simulink model "afe_abc_inv_psm_2mods"  (R2025b)
settings: Solver=ode1be  StartTime=0.0  StopTime=simlength  FixedStep=tc  MaxStep=tc
undefined symbols (not defined in the file): Adrso, afe_pwm_phase_shift_mod1, Amplitude_U, Amplitude_V, Amplitude_W, Aresd, Bresd, Cresd, Crso, CTRPIFF_CLIP_RELEASE, dead_time_AFE, dead_time_INV, deepNEGeta, deepNEGxi, deepPOSxi, emf_fb_p, emf_fb_p_ccaller_1, emf_fb_p_ccaller_2, emf_p, emf_p_ccaller_1, emf_p_ccaller_2, end_time_LVRT, fPWM_AFE, fPWM_INV, g0_161Hz, g0_500Hz, g1_161Hz, g1_500Hz, i_grid_neg_eta_lim, i_grid_neg_eta_red_lim, i_grid_neg_xi_lim, i_grid_neg_xi_red_lim, i_grid_pos_eta_lim, i_grid_pos_eta_red_lim, ibez, id_lim, ieta_neg_ref_lim, ieta_pos_ref_lim, Igrid_phase_normalization_factor, inv_pwm_phase_shift_mod1, iq_lim, ixi_pos_ref_lim, k_frt_ref, kg, ki_afe, ki_i, ki_rc_neg_grid, ki_rc_pos_grid, ki_vs, ki_w, kp_afe, kp_i, kp_rc_neg_grid, kp_rc_pos_grid, kp_vs, kp_w, kw, l1, l2, La ... (+54)
libraries: fl_lib x116, nesl_utility x62, cstblocks x14, simulink x11, single_phase_transformer_lib x3, threephase_inductor_lib x2, flexshaft_lib x1, psm x1
(part 5 of 9)

== system afe_abc_inv_psm_2mods/afe_abc_inv_psm_mod1/AFE_control/afe_control/grid_voltage_phase_lock_loops/dq_pll_ccaller ==
  ug_abc_pu : Inport
  Bus Selector : BusSelector  OutputSignals=omega_pu_hat,gamma_hat,u_grid_xi,u_grid_eta,dqpll_pll_state
  C Caller : CCaller  FunctionName=dqpll_grid_process_simulink  PortSpecificationStruct="%)30     .    N H   8    (     @         %    \"     8    !     0         %  0 \"0    $    _    07)G3F%M90  4&]R=$YA;64 4V-O<&4     26YD97@     5'EP90      4VEZ90      27-';&]B86P   X    P    !@    @    $          4    (     0    ,    !         !   P!O=70 #@   #     &    \"     0         !0    @    !     P    $         $  # &]U=  .    .     8    (    !          %    \"     $    &     0         0   ...(+3319 chars)"
  Constant : Constant  Value=ts_afe
  Data Type Conversion{1..2,4..5} (4 alike) : DataTypeConversion  OutDataTypeStr=single  SaturateOnIntegerOverflow=off  RndMeth=Floor
  Data Type Conversion{6..10} (5 alike) : DataTypeConversion  OutDataTypeStr=double  SaturateOnIntegerOverflow=off  RndMeth=Floor
  Data Type Conversion3 : DataTypeConversion  OutDataTypeStr=uint8  SaturateOnIntegerOverflow=off  RndMeth=Floor
  Demux : Demux  Outputs=3
  Quantizer1 : Quantizer  QuantizationInterval=adc_quantization
  Quantizer2 : Quantizer  QuantizationInterval=adc_quantization
  Quantizer4 : Quantizer  QuantizationInterval=adc_quantization
  Step : Step  Time=0.01  Before=1  After=0
  Unit Delay1 : UnitDelay  SampleTime=-1  HasFrameUpgradeWarning=on
  Unit Delay2 : UnitDelay  SampleTime=-1  HasFrameUpgradeWarning=on
  Unit Delay3 : UnitDelay  SampleTime=-1  HasFrameUpgradeWarning=on
  first_harmonic_tracker : Scope  NumInputPorts=3
      settings: ActiveDisplayYMinimum=-1.8038768619298935  ActiveDisplayYMaximum=1.5708545297384262
  first_harmonic_tracker_phase_u : Subsystem
  first_harmonic_tracker_phase_v : Subsystem
  first_harmonic_tracker_phase_w : Subsystem
  gamma_hat : Outport  VectorParamsAs1DForOutWhenUnconnected=off
  omega_pu_hat : Outport  Port=2  VectorParamsAs1DForOutWhenUnconnected=off
  dqpll_uxi : Outport  Port=3  VectorParamsAs1DForOutWhenUnconnected=off
  dqpll_ueta : Outport  Port=4  VectorParamsAs1DForOutWhenUnconnected=off
  dqpll_state : Outport  Port=5  VectorParamsAs1DForOutWhenUnconnected=off
  wires:
  Step/1 -> Data Type Conversion3/1
  Constant/1 -> Data Type Conversion1/1
  Data Type Conversion3/1 -> C Caller/1
  Data Type Conversion2/1 -> C Caller/2
  Data Type Conversion4/1 -> C Caller/3
  Data Type Conversion5/1 -> C Caller/4
  Data Type Conversion1/1 -> C Caller/5
  C Caller/1 -> Bus Selector/1
  Bus Selector/1 -> Data Type Conversion6/1  "<omega_pu_hat>"
  Bus Selector/2 -> Data Type Conversion7/1  "<gamma_hat>"
  Bus Selector/3 -> Data Type Conversion8/1  "<u_grid_xi>"
  Bus Selector/4 -> Data Type Conversion9/1  "<u_grid_eta>"
  Bus Selector/5 -> Data Type Conversion10/1  "<dqpll_pll_state>"
  Data Type Conversion7/1 -> gamma_hat/1
  Data Type Conversion10/1 -> dqpll_state/1
  Data Type Conversion8/1 -> dqpll_uxi/1
  Data Type Conversion9/1 -> dqpll_ueta/1
  ug_abc_pu/1 -> Demux/1
  Demux/2 -> Quantizer1/1
  Demux/1 -> Quantizer2/1
  Demux/3 -> Quantizer4/1
  Quantizer2/1 -> Unit Delay2/1
  Unit Delay2/1 -> first_harmonic_tracker_phase_u/1(u)
  Unit Delay1/1 -> first_harmonic_tracker_phase_v/1(u)
  Unit Delay3/1 -> first_harmonic_tracker_phase_w/1(u)
  Quantizer1/1 -> Unit Delay1/1
  Quantizer4/1 -> Unit Delay3/1
  Data Type Conversion6/1 -> omega_pu_hat/1
  first_harmonic_tracker_phase_u/1(u_hat) -> first_harmonic_tracker/1, Data Type Conversion2/1  "tracker_phase_u"
  first_harmonic_tracker_phase_v/1(u_hat) -> first_harmonic_tracker/2, Data Type Conversion4/1  "tracker_phase_v"
  first_harmonic_tracker_phase_w/1(u_hat) -> first_harmonic_tracker/3, Data Type Conversion5/1  "tracker_phase_w"

== system afe_abc_inv_psm_2mods/afe_abc_inv_psm_mod1/AFE_control/afe_control/grid_voltage_sequences/grid_voltage_sampling_and_alpha_beta_transformation ==
  v_abc : Inport
  Demux : Demux  Outputs=3
  Mux : Mux  Inputs=3
  sample_hold_normalization : Subsystem
  v_abc2alphabeta : MATLAB Function  TreatAsAtomicUnit=on
  u_grid_alpha : Outport
  u_grid_beta : Outport  Port=2
  tag scope: vg_abc_pu_mod1=global
  wires:
  v_abc2alphabeta/1(alpha) -> u_grid_alpha/1  "u_grid_alpha"
  v_abc2alphabeta/2(beta) -> u_grid_beta/1  "u_grid_beta"
  Demux/1 -> sample_hold_normalization/1(vg_a)
  v_abc/1 -> Demux/1
  Demux/3 -> sample_hold_normalization/3(vg_c)
  Demux/2 -> sample_hold_normalization/2(vg_b)
  sample_hold_normalization/1(vg_a_pu) -> Mux/1
  sample_hold_normalization/2(vg_b_pu) -> Mux/2
  sample_hold_normalization/3(vg_c_pu) -> Mux/3
  Mux/1 -> [vg_abc_pu_mod1], v_abc2alphabeta/1(v_abc)

== system afe_abc_inv_psm_2mods/afe_abc_inv_psm_mod1/AFE_control/afe_control/grid_voltage_sequences/v_alphabeta2xieta ==
  alpha : Inport
  beta : Inport  Port=2
  gamma : Inport  Port=3
  MATLAB Function : MATLAB Function  TreatAsAtomicUnit=on
  MATLAB Function1 : MATLAB Function  TreatAsAtomicUnit=on
  xi : Outport
  eta : Outport  Port=2
  v_grid_neg_xi : Outport  Port=3
  v_grid_neg_eta : Outport  Port=4
  wires:
  alpha/1 -> MATLAB Function1/1(alpha), MATLAB Function/1(alpha)  "u_grid_alpha"
  beta/1 -> MATLAB Function1/2(beta), MATLAB Function/2(beta)  "u_grid_beta"
  gamma/1 -> MATLAB Function1/3(gamma), MATLAB Function/3(gamma)  "gamma_grid"
  MATLAB Function/1(xi) -> xi/1  "u_grid_pos_xi"
  MATLAB Function/2(eta) -> eta/1  "u_grid_pos_eta"
  MATLAB Function1/1(xi) -> v_grid_neg_xi/1  "u_grid_neg_xi"
  MATLAB Function1/2(eta) -> v_grid_neg_eta/1  "u_grid_neg_eta"

== system afe_abc_inv_psm_2mods/afe_abc_inv_psm_mod1/AFE_control/afe_control/grid_voltage_sequences/voltage_sequence_avg ==
  v_grid_pos_xi : Inport
  v_grid_pos_eta : Inport  Port=2
  v_grid_neg_xi : Inport  Port=3
  v_grid_neg_eta : Inport  Port=4
  Variant Source{1..4} (4 alike) : VariantSource  VariantControls={use_moving_average_from_ccaller_mod1 == 1, use_moving_average_from_ccaller_mod1 == 0}
  average_filter_ccaller : Subsystem
  average_filter_simulink : Subsystem
  v_grid_pos_xi_avg : Outport
  v_grid_pos_eta_avg : Outport  Port=2
  v_grid_neg_xi_avg : Outport  Port=3
  v_grid_neg_eta_avg : Outport  Port=4
  wires:
  v_grid_pos_xi/1 -> average_filter_simulink/1(v_grid_pos_xi), average_filter_ccaller/1(v_grid_pos_xi)
  v_grid_pos_eta/1 -> average_filter_simulink/2(v_grid_pos_eta), average_filter_ccaller/2(v_grid_pos_eta)
  v_grid_neg_xi/1 -> average_filter_simulink/3(v_grid_neg_xi), average_filter_ccaller/3(v_grid_neg_xi)
  v_grid_neg_eta/1 -> average_filter_simulink/4(v_grid_neg_eta), average_filter_ccaller/4(v_grid_neg_eta)
  Variant Source4/1 -> v_grid_pos_xi_avg/1
  Variant Source1/1 -> v_grid_pos_eta_avg/1
  Variant Source2/1 -> v_grid_neg_xi_avg/1
  Variant Source3/1 -> v_grid_neg_eta_avg/1
  average_filter_ccaller/1(v_grid_pos_xi_avg) -> Variant Source4/1
  average_filter_ccaller/2(v_grid_pos_eta_avg) -> Variant Source1/1
  average_filter_ccaller/3(v_grid_neg_xi_avg) -> Variant Source2/1
  average_filter_ccaller/4(v_grid_neg_eta_avg) -> Variant Source3/1
  average_filter_simulink/1(v_grid_pos_xi_avg) -> Variant Source4/2
  average_filter_simulink/2(v_grid_pos_eta_avg) -> Variant Source1/2
  average_filter_simulink/3(v_grid_neg_xi_avg) -> Variant Source2/2
  average_filter_simulink/4(v_grid_neg_eta_avg) -> Variant Source3/2

== system afe_abc_inv_psm_2mods/afe_abc_inv_psm_mod1/INV_control/inverter_control/current_ctrl/bemf_observer ==
  ialpha_pu : Inport
  ibeta_pu : Inport  Port=2
  ualpha_pu : Inport  Port=3
  ubeta_pu : Inport  Port=4
  udc_pu : Inport  Port=5
  BEMF Observer simulink/Ccaller : Scope  NumInputPorts=2
      settings: ActiveDisplayYMinimum=-0.30362  ActiveDisplayYMaximum=1.18723
  Mux : Mux  Inputs=3
  Mux1 : Mux  Inputs=3
  Variant Source : VariantSource  VariantControls={use_observer_from_simulink_module_1 == 1, use_observer_from_ccaller_module_1 == 1}
  Variant Source1 : VariantSource  VariantControls={use_observer_from_simulink_module_1 == 1, use_observer_from_ccaller_module_1 == 1}
  bemf_observer : Subsystem
  bemf_observer_ccaller : Subsystem
  phase_fault : Subsystem  Commented=on
  tag scope: omega_hat_pu_mod1=global, theta_hat_mod1=global
  wires:
  ialpha_pu/1 -> bemf_observer/1(ialpha_pu), bemf_observer_ccaller/1(ialpha_pu)
  ibeta_pu/1 -> bemf_observer_ccaller/2(ibeta_pu), bemf_observer/2(ibeta_pu)
  Mux/1 -> BEMF Observer simulink/Ccaller/1
  Mux1/1 -> BEMF Observer simulink/Ccaller/2
  ualpha_pu/1 -> bemf_observer_ccaller/3(ualpha_pu), bemf_observer/3(ualpha_pu)
  ubeta_pu/1 -> bemf_observer_ccaller/4(ubeta_pu), bemf_observer/4(ubeta_pu)
  bemf_observer/1(omega_pu) -> Variant Source/1, Mux/1  "omega_pu"
  bemf_observer_ccaller/2(theta_hat) -> Mux1/2, Variant Source1/2  "theta_hat_code"
  bemf_observer_ccaller/1(omega_pu) -> Mux/2, Variant Source/2  "omega_pu_code"
  bemf_observer/2(theta_hat) -> Variant Source1/1, Mux1/1  "theta_hat"
  Variant Source1/1 -> [theta_hat_mod1]
  Variant Source/1 -> [omega_hat_pu_mod1]
  phase_fault/1(omega_pu_encoder) -> Mux/3
  phase_fault/2(theta_hat_encoder) -> Mux1/3
  udc_pu/1 -> bemf_observer_ccaller/5(udc_pu), bemf_observer/5(udc_pu)

== system afe_abc_inv_psm_2mods/afe_abc_inv_psm_mod1/INV_control/inverter_control/current_ctrl/current_ctrl ==
  iq_ref : Inport
  udc_pu : Inport  Port=2
  MTPA _mod1 : Subsystem
  Sqrt : Sqrt
  Square : Math  Operator=square
  Square1 : Math  Operator=square
  Sum : Sum  Inputs=|++
  dq_pi_with_vector_antiwindup mod1 : Subsystem
  id_ref _mod1 : Subsystem
      settings: PortSchema="{\"entries\":[{\"content\":{\"sides\":[{\"content\":{},\"type\":\"ConnectorPlacement.EquallySpacedRectSide\",\"uuid\":\"42af5d69-f0eb-42c6-9e03-28c1d0757323\"},{\"content\":{\"connectorIds\":[\"Out1\"],\"side\":\"RIGHT\"},\"type\":\"ConnectorPlacement.EquallySpacedRectSide\",\"uuid\":\"dd68a9f9-d15f-4e57-9d9e-130889a7b90c\"},{\"content\":{\"connectorIds\":[\"In1\"],\"side\":\"TOP\"},\"type\":\"ConnectorPlacement.EquallySpacedRectSide\",\"uuid\":\"68c797a2-8439-4b8d-8368-b7485adf0676\"}]},\"type\":\"ConnectorPlacement.EquallySpacedConnector\",\"uuid\":\"693c5f1c-0580-4626-8f13-b27865dfb3ac\"}],\"packageUris\":[\"http://schema.mathworks.com/mf0/Connector/R2020b\"],\"version\":\"1.0\"}"
  idref/id mod1 : Scope  NumInputPorts=2
      settings: ActiveDisplayYMinimum=-0.56823  ActiveDisplayYMaximum=0.06368
  iqref/iq mod1 : Scope  NumInputPorts=2
      settings: ActiveDisplayYMinimum=-1.15343  ActiveDisplayYMaximum=0.24986  DataLoggingVariableName=ScopeData2
  ud : Outport
  uq : Outport  Port=2
  tag scope: id_pu_ref_mod1=global, iq_pu_ref_mod1=global, u_mot_pu_sim_mod1=global, ud_pu_sim_mod1=global, uq_pu_sim_mod1=global
  wires:
  [iq_pu_mod1] -> iqref/iq mod1/2, dq_pi_with_vector_antiwindup mod1/4(iq)  "iq"
  [id_pu_mod1] -> idref/id mod1/2, dq_pi_with_vector_antiwindup mod1/2(id)  "id"
  MTPA _mod1/1(Id_ref_mtpa) -> id_ref _mod1/1(id_mtpa), [id_pu_ref_mod1]  "id_ref"
  iq_ref/1 -> MTPA _mod1/1(iq_ref), iqref/iq mod1/1, dq_pi_with_vector_antiwindup mod1/3(iq_ref), [iq_pu_ref_mod1]  "iq_ref"
  dq_pi_with_vector_antiwindup mod1/1(ctrl_d_u) -> ud/1, [ud_pu_sim_mod1], Square1/1
  dq_pi_with_vector_antiwindup mod1/2(ctrl_q_u) -> uq/1, [uq_pu_sim_mod1], Square/1
  Square/1 -> Sum/1
  Sum/1 -> Sqrt/1
  Square1/1 -> Sum/2
  Sqrt/1 -> [u_mot_pu_sim_mod1]
  id_ref _mod1/1(id_ref) -> idref/id mod1/1, dq_pi_with_vector_antiwindup mod1/1(id_ref)
  udc_pu/1 -> dq_pi_with_vector_antiwindup mod1/5(udc_pu)

== system afe_abc_inv_psm_2mods/afe_abc_inv_psm_mod1/INV_control/inverter_control/current_ctrl/current_transformation ==
  u : Inport
  v : Inport  Port=2
  w : Inport  Port=3
  alphabeta2dq : MATLAB Function  TreatAsAtomicUnit=on
  uvw2alphabeta : MATLAB Function  TreatAsAtomicUnit=on
  tag scope: ialpha_pu_mod1=global, ibeta_pu_mod1=global, id_pu_mod1=global, iq_pu_mod1=global
  wires:
  w/1 -> uvw2alphabeta/3(w)
  alphabeta2dq/2(q) -> [iq_pu_mod1]  "iq_pu"
  alphabeta2dq/1(d) -> [id_pu_mod1]  "id_pu"
  v/1 -> uvw2alphabeta/2(v)
  uvw2alphabeta/2(beta) -> [ibeta_pu_mod1], alphabeta2dq/2(beta)  "ibeta_pu"
  uvw2alphabeta/1(alpha) -> [ialpha_pu_mod1], alphabeta2dq/1(alpha)  "ialpha_pu"
  [theta_hat_mod1] -> alphabeta2dq/3(gamma)
  u/1 -> uvw2alphabeta/1(u)

== system afe_abc_inv_psm_2mods/afe_abc_inv_psm_mod1/INV_control/inverter_control/current_ctrl/sample_hold_normalization ==
  iu : Inport
  iv : Inport  Port=2
  iw : Inport  Port=3
  Gain3 : Gain  Gain=-1
  Gain4 : Gain  Gain=-1
  Gain5 : Gain  Gain=-1
  Quantizer1 : Quantizer  QuantizationInterval=adc_quantization
  Quantizer2 : Quantizer  QuantizationInterval=adc_quantization
  Quantizer4 : Quantizer  QuantizationInterval=adc_quantization
  Unit Delay : UnitDelay  SampleTime=-1  HasFrameUpgradeWarning=on
  Unit Delay1 : UnitDelay  SampleTime=-1  HasFrameUpgradeWarning=on
  Unit Delay4 : UnitDelay  SampleTime=-1  HasFrameUpgradeWarning=on
  iu_pu : Outport
  iv_pu : Outport  Port=2
  iw_pu : Outport  Port=3
  wires:
  Unit Delay4/1 -> Gain5/1
  Unit Delay1/1 -> Gain4/1
  Unit Delay/1 -> Gain3/1
  Quantizer4/1 -> Unit Delay/1
  Quantizer1/1 -> Unit Delay1/1
  Quantizer2/1 -> Unit Delay4/1
  iu/1 -> Quantizer4/1
  iv/1 -> Quantizer1/1
  iw/1 -> Quantizer2/1
  Gain3/1 -> iu_pu/1
  Gain4/1 -> iv_pu/1
  Gain5/1 -> iw_pu/1

== system afe_abc_inv_psm_2mods/afe_abc_inv_psm_mod1/afe/sv_pwm/modulator1/PWM generator ==
  time_source : Inport
  phase : Inport  Port=2
  m_uvw() : Inport  Port=3
  Constant8 : Constant  Value=tc
  Constant9 : Constant  Value=f
  MATLAB Function : MATLAB Function  TreatAsAtomicUnit=on  SystemSampleTime=tc
  MATLAB Function1 : MATLAB Function  TreatAsAtomicUnit=on  SystemSampleTime=tc
  gate commands : Subsystem
  period : Constant  Value=1/f
  trgo : Outport
  gate_cmds : Outport  Port=2
  wires:
  period/1 -> MATLAB Function/3(period)
  phase/1 -> MATLAB Function/2(phase)
  MATLAB Function/1(y) -> gate commands/1(ramp_up_down), MATLAB Function1/3(ramp_up_down)
  MATLAB Function1/1(trgo) -> trgo/1
  Constant8/1 -> MATLAB Function1/1(sampling_time)
  Constant9/1 -> MATLAB Function1/2(fPWM)
  m_uvw()/1 -> gate commands/2(m_uvw())
  gate commands/1(gate_cmds) -> gate_cmds/1
  time_source/1 -> MATLAB Function/1(t)

== system afe_abc_inv_psm_2mods/afe_abc_inv_psm_mod1/inverter/inverter/sv_pwm/modulator1 ==
  u : Inport
  v : Inport  Port=2
  w : Inport  Port=3
  phase : Inport  Port=4
  Bus Creator : BusCreator  Inputs=3
  PWM generator : Subsystem  mask{f=fPWM_INV, m_up=0.98, m_low=0.02, dead_time=dead_time_INV, pos_cmd_gate=15, neg_cmd_gate=-10, polarity=1, tc=tc}
      mask prompts: f "Frequency (Hz)"; m_up "Max Input Modulation Value"; m_low "Min Input Modulation Value"; dead_time "Dead Time (s)"; pos_cmd_gate "Positive Gate Voltage (V)"; neg_cmd_gate "Negative Gate Voltage (V)"; polarity "Polarity (pu)"; tc "Sampling time"
  gate_cmds : Outport
  tag scope: TRGO_inv_module_1=global
  wires:
  [time_inv_module_1] -> PWM generator/1(time_source)
  Bus Creator/1 -> PWM generator/3(m_uvw())
  PWM generator/1(trgo) -> [TRGO_inv_module_1]
  u/1 -> Bus Creator/1
  v/1 -> Bus Creator/2
  w/1 -> Bus Creator/3
  phase/1 -> PWM generator/2(phase)
  PWM generator/2(gate_cmds) -> gate_cmds/1

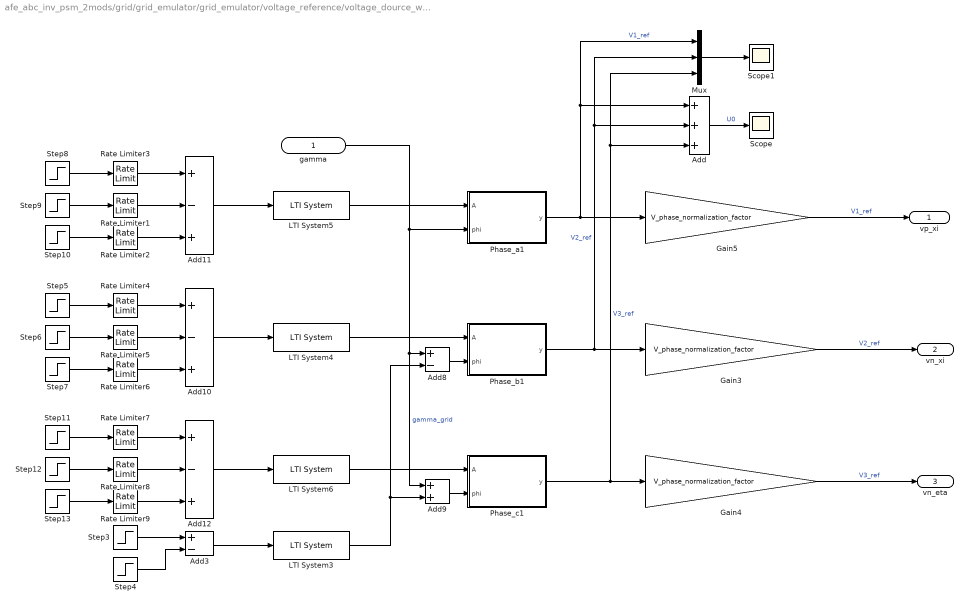
== system afe_abc_inv_psm_2mods/grid/grid_emulator/grid_emulator/voltage_reference/voltage_dource_with_frt ==
  gamma : Inport
  Add : Sum  Inputs=+++
  Add10 : Sum  Inputs=+-+
  Add11 : Sum  Inputs=+-+
  Add12 : Sum  Inputs=+-+
  Add3 : Sum  Inputs=+-
  Add8 : Sum  Inputs=+-
  Add9 : Sum
  Gain3 : Gain  Gain=V_phase_normalization_factor
  Gain4 : Gain  Gain=V_phase_normalization_factor
  Gain5 : Gain  Gain=V_phase_normalization_factor
  LTI System{3..6} (4 alike) : cstblocks/LTI System  sys=LVRT_flt_ss_c  IC=[0]  PadeOrder=0
  Mux : Mux  Inputs=3
  Phase_a1 : MATLAB Function  TreatAsAtomicUnit=on
  Phase_b1 : MATLAB Function  TreatAsAtomicUnit=on
  Phase_c1 : MATLAB Function  TreatAsAtomicUnit=on
  Rate Limiter{1..9} (9 alike) : RateLimiter  RisingSlewLimit=Vemu_ref_norm/t_ramp  FallingSlewLimit=-Vemu_ref_norm/t_ramp  SampleTimeMode=inherited
  Scope : Scope
      settings: ActiveDisplayYMinimum=-1E-15  ActiveDisplayYMaximum=8E-16
  Scope1 : Scope
      settings: ActiveDisplayYMinimum=-1.25511  ActiveDisplayYMaximum=1.25511
  Step10 : Step  Time=end_time_LVRT  After=Vemu_ref_norm*(1-Amplitude_U)  SampleTime=0
  Step11 : Step  Time=0  After=Vemu_ref_norm  SampleTime=0
  Step12 : Step  Time=start_time_LVRT  After=Vemu_ref_norm*(1-Amplitude_W)  SampleTime=0
  Step13 : Step  Time=end_time_LVRT  After=Vemu_ref_norm*(1-Amplitude_W)  SampleTime=0
  Step3 : Step  Time=start_time_LVRT  After=Phase_shift  SampleTime=0
  Step4 : Step  Time=end_time_LVRT  After=Phase_shift  SampleTime=0
  Step5 : Step  Time=0  After=Vemu_ref_norm  SampleTime=0
  Step6 : Step  Time=start_time_LVRT  After=Vemu_ref_norm*(1-Amplitude_V)  SampleTime=0
  Step7 : Step  Time=end_time_LVRT  After=Vemu_ref_norm*(1-Amplitude_V)  SampleTime=0
  Step8 : Step  Time=0  After=Vemu_ref_norm  SampleTime=0
  Step9 : Step  Time=start_time_LVRT  After=Vemu_ref_norm*(1-Amplitude_U)  SampleTime=0
  vp_xi : Outport  VectorParamsAs1DForOutWhenUnconnected=off
  vn_xi : Outport  Port=2  VectorParamsAs1DForOutWhenUnconnected=off
  vn_eta : Outport  Port=3  VectorParamsAs1DForOutWhenUnconnected=off
  wires:
  Phase_c1/1(y) -> Mux/3, Add/3, Gain4/1  "V3_ref"
  LTI System6/1 -> Phase_c1/1(A)
  gamma/1 -> Add9/1, Add8/1, Phase_a1/2(phi)  "gamma_grid"
  Add9/1 -> Phase_c1/2(phi)
  Add8/1 -> Phase_b1/2(phi)
  Phase_b1/1(y) -> Mux/2, Add/2, Gain3/1  "V2_ref"
  Phase_a1/1(y) -> Mux/1, Add/1, Gain5/1  "V1_ref"
  LTI System4/1 -> Phase_b1/1(A)
  Step5/1 -> Rate Limiter4/1
  Step6/1 -> Rate Limiter5/1
  Step7/1 -> Rate Limiter6/1
  Add10/1 -> LTI System4/1
  Step8/1 -> Rate Limiter3/1
  Add11/1 -> LTI System5/1
  Step9/1 -> Rate Limiter1/1
  Step10/1 -> Rate Limiter2/1
  LTI System5/1 -> Phase_a1/1(A)
  Add12/1 -> LTI System6/1
  Rate Limiter3/1 -> Add11/1
  Rate Limiter1/1 -> Add11/2
  Rate Limiter2/1 -> Add11/3
  Rate Limiter4/1 -> Add10/1
  Rate Limiter5/1 -> Add10/2
  Rate Limiter6/1 -> Add10/3
  Step12/1 -> Rate Limiter8/1
  Rate Limiter8/1 -> Add12/2
  Step13/1 -> Rate Limiter9/1
  Rate Limiter9/1 -> Add12/3
  Step11/1 -> Rate Limiter7/1
  Rate Limiter7/1 -> Add12/1
  Gain5/1 -> vp_xi/1  "V1_ref"
  Gain3/1 -> vn_xi/1  "V2_ref"
  Gain4/1 -> vn_eta/1  "V3_ref"
  Add3/1 -> LTI System3/1
  Step3/1 -> Add3/1
  Step4/1 -> Add3/2
  LTI System3/1 -> Add9/2, Add8/2
  Add/1 -> Scope/1  "U0"
  Mux/1 -> Scope1/1

== system afe_abc_inv_psm_2mods/afe_abc_inv_psm_mod1/AFE_control/afe_control/FRT-VDE4110/FRT-Detection/dvxi_n//dt ==
  x : Inport
  Gain : Gain  Gain=l1
  Gain1 : Gain  Gain=l2
  Gain5 : Gain  Gain=ts_afe
  Sum : Sum  Inputs=-+|
  Sum1 : Sum  Inputs=|++
  Sum2 : Sum  Inputs=|++
  Sum8 : Sum  Inputs=++|
  Unit Delay1 : UnitDelay  SampleTime=-1  HasFrameUpgradeWarning=on
  Unit Delay2 : UnitDelay  SampleTime=-1  HasFrameUpgradeWarning=on
  xdot_hat : Outport  VectorParamsAs1DForOutWhenUnconnected=off
  wires:
  Sum8/1 -> Unit Delay1/1
  Sum/1 -> Gain/1, Gain1/1
  Unit Delay1/1 -> Sum/1, Sum2/2  "x_hat"
  Sum2/1 -> Sum8/2
  Unit Delay2/1 -> Gain5/1, Sum1/2, xdot_hat/1
  Gain/1 -> Sum1/1
  Sum1/1 -> Unit Delay2/1
  Gain5/1 -> Sum8/1
  x/1 -> Sum/2  "x"
  Gain1/1 -> Sum2/1

== system afe_abc_inv_psm_2mods/afe_abc_inv_psm_mod1/AFE_control/afe_control/FRT-VDE4110/FRT-Detection/dvxi_p//dt ==
  x : Inport
  Gain : Gain  Gain=l1
  Gain1 : Gain  Gain=l2
  Gain5 : Gain  Gain=ts_afe
  Sum : Sum  Inputs=-+|
  Sum1 : Sum  Inputs=|++
  Sum2 : Sum  Inputs=|++
  Sum8 : Sum  Inputs=++|
  Unit Delay1 : UnitDelay  SampleTime=-1  HasFrameUpgradeWarning=on
  Unit Delay2 : UnitDelay  SampleTime=-1  HasFrameUpgradeWarning=on
  xdot_hat : Outport  VectorParamsAs1DForOutWhenUnconnected=off
  wires:
  Gain1/1 -> Sum2/1
  x/1 -> Sum/2  "x"
  Gain5/1 -> Sum8/1
  Sum1/1 -> Unit Delay2/1
  Gain/1 -> Sum1/1
  Sum2/1 -> Sum8/2
  Unit Delay1/1 -> Sum2/2, Sum/1  "x_hat"
  Sum/1 -> Gain1/1, Gain/1
  Sum8/1 -> Unit Delay1/1
  Unit Delay2/1 -> xdot_hat/1, Sum1/2, Gain5/1

== system afe_abc_inv_psm_2mods/afe_abc_inv_psm_mod1/AFE_control/afe_control/FRT-VDE4110/FRT-PosNegReactiveCurrentReferences/avg_flt_500ms ==
  In1 : Inport
  Constant : Constant  Value=2*pi/500e-3
  Constant1 : Constant  Value=ts_afe
  Constant2 : Constant
  Sum : Sum  Inputs=|-+
  avg_flt_1 : MATLAB Function  TreatAsAtomicUnit=on
  Out1 : Outport  VectorParamsAs1DForOutWhenUnconnected=off
  wires:
  avg_flt_1/1(y1) -> Out1/1  "output"
  Constant1/1 -> avg_flt_1/3(ts)
  Constant/1 -> avg_flt_1/2(w)
  In1/1 -> avg_flt_1/1(x)  "input"
  Constant2/1 -> Sum/2
  [frt_active_mod1] -> Sum/1
  Sum/1 -> avg_flt_1/4(enable)

== system afe_abc_inv_psm_2mods/afe_abc_inv_psm_mod1/AFE_control/afe_control/FRT-VDE4110/FRT-PosNegReactiveCurrentReferences/avg_flt_500ms1 ==
  In1 : Inport
  Constant : Constant  Value=2*pi/500e-3
  Constant1 : Constant  Value=ts_afe
  Constant2 : Constant
  Sum : Sum  Inputs=|-+
  avg_flt_1 : MATLAB Function  TreatAsAtomicUnit=on
  Out1 : Outport  VectorParamsAs1DForOutWhenUnconnected=off
  wires:
  Sum/1 -> avg_flt_1/4(enable)
  [frt_active_mod1] -> Sum/1
  Constant2/1 -> Sum/2
  In1/1 -> avg_flt_1/1(x)  "input"
  Constant/1 -> avg_flt_1/2(w)
  Constant1/1 -> avg_flt_1/3(ts)
  avg_flt_1/1(y1) -> Out1/1  "output"

== system afe_abc_inv_psm_2mods/afe_abc_inv_psm_mod1/AFE_control/afe_control/FRT-VDE4110/FRT-PosNegReactiveCurrentReferences/avg_flt_500ms2 ==
  In1 : Inport
  Constant : Constant  Value=2*pi/500e-3
  Constant1 : Constant  Value=ts_afe
  Constant2 : Constant
  Sum : Sum  Inputs=|-+
  avg_flt_1 : MATLAB Function  TreatAsAtomicUnit=on
  Out1 : Outport  VectorParamsAs1DForOutWhenUnconnected=off
  wires:
  avg_flt_1/1(y1) -> Out1/1  "output"
  Constant1/1 -> avg_flt_1/3(ts)
  Constant/1 -> avg_flt_1/2(w)
  In1/1 -> avg_flt_1/1(x)  "input"
  Constant2/1 -> Sum/2
  [frt_active_mod1] -> Sum/1
  Sum/1 -> avg_flt_1/4(enable)

== system afe_abc_inv_psm_2mods/afe_abc_inv_psm_mod1/AFE_control/afe_control/FRT-VDE4110/FRT-PosNegReactiveCurrentReferences/avg_flt_500ms3 ==
  In1 : Inport
  Constant : Constant  Value=2*pi/500e-3
  Constant1 : Constant  Value=ts_afe
  Constant2 : Constant
  Sum : Sum  Inputs=|-+
  avg_flt_1 : MATLAB Function  TreatAsAtomicUnit=on
  Out1 : Outport  VectorParamsAs1DForOutWhenUnconnected=off
  wires:
  Sum/1 -> avg_flt_1/4(enable)
  [frt_active_mod1] -> Sum/1
  Constant2/1 -> Sum/2
  In1/1 -> avg_flt_1/1(x)  "input"
  Constant/1 -> avg_flt_1/2(w)
  Constant1/1 -> avg_flt_1/3(ts)
  avg_flt_1/1(y1) -> Out1/1  "output"

== system afe_abc_inv_psm_2mods/afe_abc_inv_psm_mod1/AFE_control/afe_control/FRT-VDE4110/FRT-PosNegReactiveCurrentReferences/u_161Hz_flt1 ==
  input : Inport
  Gain3 : Gain  Gain=g1_161Hz
  Gain6 : Gain  Gain=g0_161Hz
  Sum : Sum  Inputs=|++
  Unit Delay1 : UnitDelay  SampleTime=-1  HasFrameUpgradeWarning=on
  output : Outport  VectorParamsAs1DForOutWhenUnconnected=off
  wires:
  Gain6/1 -> Sum/1
  input/1 -> Gain6/1
  Unit Delay1/1 -> Gain3/1
  Gain3/1 -> Sum/2
  Sum/1 -> Unit Delay1/1, output/1

== system afe_abc_inv_psm_2mods/afe_abc_inv_psm_mod1/AFE_control/afe_control/FRT-VDE4110/FRT-PosNegReactiveCurrentReferences/u_161Hz_flt2 ==
  input : Inport
  Gain3 : Gain  Gain=g1_161Hz
  Gain6 : Gain  Gain=g0_161Hz
  Sum : Sum  Inputs=|++
  Unit Delay1 : UnitDelay  SampleTime=-1  HasFrameUpgradeWarning=on
  output : Outport  VectorParamsAs1DForOutWhenUnconnected=off
  wires:
  Sum/1 -> output/1, Unit Delay1/1
  Gain3/1 -> Sum/2
  Unit Delay1/1 -> Gain3/1
  input/1 -> Gain6/1
  Gain6/1 -> Sum/1

== system afe_abc_inv_psm_2mods/afe_abc_inv_psm_mod1/AFE_control/afe_control/FRT-VDE4110/FRT-PosNegReactiveCurrentReferences/u_161Hz_flt3 ==
  input : Inport
  Gain3 : Gain  Gain=g1_161Hz
  Gain6 : Gain  Gain=g0_161Hz
  Sum : Sum  Inputs=|++
  Unit Delay1 : UnitDelay  SampleTime=-1  HasFrameUpgradeWarning=on
  output : Outport  VectorParamsAs1DForOutWhenUnconnected=off
  wires:
  Gain6/1 -> Sum/1
  input/1 -> Gain6/1
  Unit Delay1/1 -> Gain3/1
  Gain3/1 -> Sum/2
  Sum/1 -> Unit Delay1/1, output/1

== system afe_abc_inv_psm_2mods/afe_abc_inv_psm_mod1/AFE_control/afe_control/current_ctrl/Inner Loop Current Control/Current-Control, Phase a ==
  In1 : Inport
  In2 : Inport  Port=2
  Add : Sum
  Cresd./Tcontrol new1 : Gain  Gain=Cresd  Multiplication=Matrix(K*u)
  Gain : Gain  Gain=kp_afe
  Gain1 : Gain  Gain=ki_afe
  Gain2 : Gain  Gain=Bresd  Multiplication=Matrix(K*u)
  Gain3 : Gain  Gain=Aresd  Multiplication=Matrix(K*u)
  Sum : Sum  Inputs=|+-
  Sum2 : Sum  Inputs=|++  SaturateOnIntegerOverflow=on
  Unit Delay : UnitDelay  InitialCondition=[0 0]  SampleTime=-1  HasFrameUpgradeWarning=on
  Out1 : Outport
  wires:
  In1/1 -> Sum/1  "isa_ref"
  In2/1 -> Sum/2  "isa"
  Add/1 -> Out1/1  "v_a"
  Sum/1 -> Gain1/1, Gain/1
  Gain/1 -> Add/1
  Gain1/1 -> Gain2/1  "u(k)"
  Gain2/1 -> Sum2/1
  Unit Delay/1 -> Gain3/1, Cresd./Tcontrol new1/1  "x(k)"
  Sum2/1 -> Unit Delay/1  "x(k+1)"
  Gain3/1 -> Sum2/2
  Cresd./Tcontrol new1/1 -> Add/2  "y(k)"

== system afe_abc_inv_psm_2mods/afe_abc_inv_psm_mod1/AFE_control/afe_control/current_ctrl/Inner Loop Current Control/Current-Control, Phase b ==
  In1 : Inport
  In2 : Inport  Port=2
  Add : Sum
  Cresd./Tcontrol new1 : Gain  Gain=Cresd  Multiplication=Matrix(K*u)
  Gain : Gain  Gain=kp_afe
  Gain1 : Gain  Gain=ki_afe
  Gain2 : Gain  Gain=Bresd  Multiplication=Matrix(K*u)
  Gain3 : Gain  Gain=Aresd  Multiplication=Matrix(K*u)
  Sum : Sum  Inputs=|+-
  Sum2 : Sum  Inputs=|++  SaturateOnIntegerOverflow=on
  Unit Delay : UnitDelay  InitialCondition=[0 0]  SampleTime=-1  HasFrameUpgradeWarning=on
  Out1 : Outport
  wires:
  Cresd./Tcontrol new1/1 -> Add/2  "y(k)"
  Gain3/1 -> Sum2/2
  Sum2/1 -> Unit Delay/1  "x(k+1)"
  Unit Delay/1 -> Cresd./Tcontrol new1/1, Gain3/1  "x(k)"
  Gain2/1 -> Sum2/1
  Gain1/1 -> Gain2/1  "u(k)"
  Gain/1 -> Add/1
  Sum/1 -> Gain/1, Gain1/1
  Add/1 -> Out1/1  "v_a"
  In2/1 -> Sum/2  "isb"
  In1/1 -> Sum/1  "isb_ref"

== system afe_abc_inv_psm_2mods/afe_abc_inv_psm_mod1/AFE_control/afe_control/current_ctrl/Inner Loop Current Control/Current-Control, Phase c ==
  In1 : Inport
  In2 : Inport  Port=2
  Add : Sum
  Cresd./Tcontrol new1 : Gain  Gain=Cresd  Multiplication=Matrix(K*u)
  Gain : Gain  Gain=kp_afe
  Gain1 : Gain  Gain=ki_afe
  Gain2 : Gain  Gain=Bresd  Multiplication=Matrix(K*u)
  Gain3 : Gain  Gain=Aresd  Multiplication=Matrix(K*u)
  Sum : Sum  Inputs=|+-
  Sum2 : Sum  Inputs=|++  SaturateOnIntegerOverflow=on
  Unit Delay : UnitDelay  InitialCondition=[0 0]  SampleTime=-1  HasFrameUpgradeWarning=on
  Out1 : Outport
  wires:
  In1/1 -> Sum/1  "isc_ref"
  In2/1 -> Sum/2  "isc"
  Add/1 -> Out1/1  "v_a"
  Sum/1 -> Gain1/1, Gain/1
  Gain/1 -> Add/1
  Gain1/1 -> Gain2/1  "u(k)"
  Gain2/1 -> Sum2/1
  Unit Delay/1 -> Gain3/1, Cresd./Tcontrol new1/1  "x(k)"
  Sum2/1 -> Unit Delay/1  "x(k+1)"
  Gain3/1 -> Sum2/2
  Cresd./Tcontrol new1/1 -> Add/2  "y(k)"

== system afe_abc_inv_psm_2mods/afe_abc_inv_psm_mod1/AFE_control/afe_control/grid_current_sequences_and_reactive_pwr_ctrl/current_sequence_avg/average_filter_ccaller ==
  i_grid_pos_xi : Inport
  i_grid_pos_eta : Inport  Port=2
  i_grid_neg_xi : Inport  Port=3
  i_grid_neg_eta : Inport  Port=4
  Moving Average Filter1 : Subsystem
  Moving Average Filter2 : Subsystem
  Moving Average Filter3 : Subsystem
  Moving Average Filter5 : Subsystem
  i_grid_pos_xi_avg : Outport
  i_grid_pos_eta_avg : Outport  Port=2
  i_grid_neg_xi_avg : Outport  Port=3
  i_grid_neg_eta_avg : Outport  Port=4
  wires:
  Moving Average Filter1/1(xi) -> i_grid_pos_eta_avg/1
  [omega_grid_pll_mod1] -> Moving Average Filter5/2(In3), Moving Average Filter1/2(In3), Moving Average Filter3/2(In3), Moving Average Filter2/2(In3)
  i_grid_pos_eta/1 -> Moving Average Filter1/1(In2)
  Moving Average Filter3/1(xi) -> i_grid_neg_eta_avg/1
  i_grid_neg_xi/1 -> Moving Average Filter2/1(In2)
  Moving Average Filter2/1(xi) -> i_grid_neg_xi_avg/1
  i_grid_pos_xi/1 -> Moving Average Filter5/1(In2)
  i_grid_neg_eta/1 -> Moving Average Filter3/1(In2)
  Moving Average Filter5/1(xi) -> i_grid_pos_xi_avg/1

== system afe_abc_inv_psm_2mods/afe_abc_inv_psm_mod1/AFE_control/afe_control/grid_current_sequences_and_reactive_pwr_ctrl/current_sequence_avg/average_filter_simulink ==
  i_grid_pos_xi : Inport
  i_grid_pos_eta : Inport  Port=2
  i_grid_neg_xi : Inport  Port=3
  i_grid_neg_eta : Inport  Port=4
  moving_avarage_1 : Subsystem
  moving_avarage_2 : Subsystem
  moving_avarage_3 : Subsystem
  moving_avarage_4 : Subsystem
  i_grid_pos_xi_avg : Outport
  i_grid_pos_eta_avg : Outport  Port=2
  i_grid_neg_xi_avg : Outport  Port=3
  i_grid_neg_eta_avg : Outport  Port=4
  wires:
  i_grid_neg_xi/1 -> moving_avarage_3/1(in)
  i_grid_pos_xi/1 -> moving_avarage_1/1(in)
  i_grid_neg_eta/1 -> moving_avarage_4/1(in)
  i_grid_pos_eta/1 -> moving_avarage_2/1(in)
  moving_avarage_1/1(out) -> i_grid_pos_xi_avg/1
  moving_avarage_2/1(out) -> i_grid_pos_eta_avg/1
  moving_avarage_3/1(out) -> i_grid_neg_xi_avg/1
  moving_avarage_4/1(out) -> i_grid_neg_eta_avg/1

== system afe_abc_inv_psm_2mods/afe_abc_inv_psm_mod1/AFE_control/afe_control/grid_current_sequences_and_reactive_pwr_ctrl/grid_current_sampling_and_alpha_beta_transformation/sample_hold_normalization ==
  ig_a : Inport
  ig_b : Inport  Port=2
  ig_c : Inport  Port=3
  Gain4 : Gain  Gain=-1
  Gain5 : Gain  Gain=-1
  Gain6 : Gain  Gain=-1
  Quantizer1 : Quantizer  QuantizationInterval=adc_quantization
  Quantizer2 : Quantizer  QuantizationInterval=adc_quantization
  Quantizer4 : Quantizer  QuantizationInterval=adc_quantization
  Unit Delay : UnitDelay  SampleTime=-1  HasFrameUpgradeWarning=on
  Unit Delay1 : UnitDelay  SampleTime=-1  HasFrameUpgradeWarning=on
  Unit Delay2 : UnitDelay  SampleTime=-1  HasFrameUpgradeWarning=on
  ig_a_pu : Outport
  ig_b_pu : Outport  Port=2
  ig_c_pu : Outport  Port=3
  wires:
  Quantizer1/1 -> Unit Delay1/1
  Quantizer4/1 -> Unit Delay/1
  Quantizer2/1 -> Unit Delay2/1
  ig_a/1 -> Quantizer4/1
  ig_b/1 -> Quantizer1/1
  ig_c/1 -> Quantizer2/1
  Unit Delay/1 -> Gain4/1
  Unit Delay1/1 -> Gain5/1
  Unit Delay2/1 -> Gain6/1
  Gain4/1 -> ig_a_pu/1
  Gain5/1 -> ig_b_pu/1
  Gain6/1 -> ig_c_pu/1

== system afe_abc_inv_psm_2mods/afe_abc_inv_psm_mod1/AFE_control/afe_control/grid_current_sequences_and_reactive_pwr_ctrl/sequences_current_control/Negative-Seq. eta-Control ==
  ff : Inport
  e : Inport  Port=2
  1/Ti : Gain  Gain=kp_rc_neg_grid  SaturateOnIntegerOverflow=on  OutDataTypeStr=Inherit: Same as input  ParamDataTypeStr=Inherit: Same as input
  Saturation : Saturate  UpperLimit=ieta_neg_ref_lim  LowerLimit=-ieta_neg_ref_lim
  Sum : Sum  Inputs=|++
  Sum2 : Sum  Inputs=+++  SaturateOnIntegerOverflow=on
  Sum3 : Sum  Inputs=-+  SaturateOnIntegerOverflow=on
  Unit Delay4 : UnitDelay  SampleTime=-1  HasFrameUpgradeWarning=on
  kp : Gain  Gain=ki_rc_neg_grid*ts_afe  SaturateOnIntegerOverflow=on  OutDataTypeStr=Inherit: Same as input  ParamDataTypeStr=Inherit: Same as input
  u : Outport  VectorParamsAs1DForOutWhenUnconnected=off
  wires:
  Unit Delay4/1 -> Sum2/3
  Sum3/1 -> Unit Delay4/1
  kp/1 -> Sum2/2
  Sum2/1 -> Saturation/1
  1/Ti/1 -> Sum2/1, Sum3/1
  Saturation/1 -> Sum/1, Sum3/2
  Sum/1 -> u/1
  e/1 -> 1/Ti/1, kp/1  "e"
  ff/1 -> Sum/2

== system afe_abc_inv_psm_2mods/afe_abc_inv_psm_mod1/AFE_control/afe_control/grid_current_sequences_and_reactive_pwr_ctrl/sequences_current_control/Negative-Seq. xi-Control ==
  ff : Inport
  e : Inport  Port=2
  1/Ti : Gain  Gain=kp_rc_neg_grid  SaturateOnIntegerOverflow=on  OutDataTypeStr=Inherit: Same as input  ParamDataTypeStr=Inherit: Same as input
  Saturation : Saturate  UpperLimit=ieta_pos_ref_lim  LowerLimit=-ieta_pos_ref_lim
  Sum : Sum  Inputs=|++
  Sum2 : Sum  Inputs=+++  SaturateOnIntegerOverflow=on
  Sum3 : Sum  Inputs=-+  SaturateOnIntegerOverflow=on
  Unit Delay4 : UnitDelay  SampleTime=-1  HasFrameUpgradeWarning=on
  kp : Gain  Gain=ki_rc_neg_grid*ts_afe  SaturateOnIntegerOverflow=on  OutDataTypeStr=Inherit: Same as input  ParamDataTypeStr=Inherit: Same as input
  u : Outport  VectorParamsAs1DForOutWhenUnconnected=off
  wires:
  Unit Delay4/1 -> Sum2/3
  Sum3/1 -> Unit Delay4/1
  kp/1 -> Sum2/2
  Sum2/1 -> Saturation/1
  1/Ti/1 -> Sum2/1, Sum3/1
  Saturation/1 -> Sum/1, Sum3/2
  Sum/1 -> u/1
  e/1 -> 1/Ti/1, kp/1  "e"
  ff/1 -> Sum/2

== system afe_abc_inv_psm_2mods/afe_abc_inv_psm_mod1/AFE_control/afe_control/grid_current_sequences_and_reactive_pwr_ctrl/sequences_current_control/Positive-Seq. eta-Control ==
  ff : Inport
  e : Inport  Port=2
  1/Ti : Gain  Gain=kp_rc_pos_grid  SaturateOnIntegerOverflow=on  OutDataTypeStr=Inherit: Same as input  ParamDataTypeStr=Inherit: Same as input
  Saturation : Saturate  UpperLimit=ieta_pos_ref_lim  LowerLimit=-ieta_pos_ref_lim
  Sum : Sum  Inputs=|++
  Sum2 : Sum  Inputs=+++  SaturateOnIntegerOverflow=on
  Sum3 : Sum  Inputs=-+  SaturateOnIntegerOverflow=on
  Unit Delay4 : UnitDelay  SampleTime=-1  HasFrameUpgradeWarning=on
  kp : Gain  Gain=ki_rc_pos_grid*ts_afe  SaturateOnIntegerOverflow=on  OutDataTypeStr=Inherit: Same as input  ParamDataTypeStr=Inherit: Same as input
  u : Outport  VectorParamsAs1DForOutWhenUnconnected=off
  wires:
  Unit Delay4/1 -> Sum2/3
  Sum3/1 -> Unit Delay4/1
  kp/1 -> Sum2/2
  Sum2/1 -> Saturation/1
  1/Ti/1 -> Sum2/1, Sum3/1
  Saturation/1 -> Sum/1, Sum3/2
  Sum/1 -> u/1
  e/1 -> 1/Ti/1, kp/1  "e"
  ff/1 -> Sum/2

== system afe_abc_inv_psm_2mods/afe_abc_inv_psm_mod1/AFE_control/afe_control/grid_voltage_phase_lock_loops/DDSRF-PLL/pll_stageA ==
  gamma_grid : Inport
  ug_abc_pu : Inport  Port=2
  Demux : Demux  Outputs=3
  Math Function : Math  Operator=magnitude^2  SignedPower=on
  Math Function1 : Math  Operator=magnitude^2  SignedPower=on
  Reciprocal Sqrt : Sqrt  Operator=rSqrt
  Saturation : Saturate  UpperLimit=inf  LowerLimit=0.02
  Sum : Sum  Inputs=|++
  mormalization_and_transformation : Subsystem
  sequences : Subsystem
  u_grid_pos_xi : Outport  VectorParamsAs1DForOutWhenUnconnected=off
  u_grid_pos_eta : Outport  Port=2  VectorParamsAs1DForOutWhenUnconnected=off
  tag scope: Vgrid_unorm=global
  wires:
  Saturation/1 -> Reciprocal Sqrt/1
  Reciprocal Sqrt/1 -> [Vgrid_unorm]
  Sum/1 -> Saturation/1
  Math Function1/1 -> Sum/2
  Math Function/1 -> Sum/1
  mormalization_and_transformation/2(ug_beta) -> sequences/2(u_grid_beta), Math Function1/1
  mormalization_and_transformation/1(ug_alpha) -> sequences/1(u_grid_alpha), Math Function/1
  Demux/3 -> mormalization_and_transformation/3(ug_c)
  Demux/2 -> mormalization_and_transformation/2(ug_b)
  Demux/1 -> mormalization_and_transformation/1(ug_a)
  ug_abc_pu/1 -> Demux/1
  sequences/1(u_grid_pos_xi) -> u_grid_pos_xi/1
  sequences/2(u_grid_pos_eta) -> u_grid_pos_eta/1
  gamma_grid/1 -> sequences/3(phase_angle)

== system afe_abc_inv_psm_2mods/afe_abc_inv_psm_mod1/AFE_control/afe_control/grid_voltage_phase_lock_loops/DDSRF-PLL/pll_stageB ==
  u_grid_pos_xi : Inport
  u_grid_pos_eta : Inport  Port=2
  -2<x<2 : Saturate  UpperLimit=2  LowerLimit=-2
  Constant2 : Constant
  Constant3 : Constant  Value=0
  Constant4 : Constant  Value=omega_grid_nom
  Constant5 : Constant
  Constant6 : Constant  Value=-1
  Math Function : Math  Operator=magnitude^2  SignedPower=on
  Math Function2 : Math  Operator=magnitude^2  SignedPower=on
  Product{,1..3} (4 alike) : Product  RndMeth=Zero
  Sqrt : Sqrt
  Sum : Sum  Inputs=|-+
  Sum1 : Sum  Inputs=|-+
  Sum2 : Sum  Inputs=|++
  Sum3 : Sum  SaturateOnIntegerOverflow=on
  Sum4 : Sum  SaturateOnIntegerOverflow=on
  Sum5 : Sum  Inputs=++|
  Switch : Switch  Criteria=u2 > Threshold  SaturateOnIntegerOverflow=off  InputSameDT=off
  To Workspace5 : ToWorkspace  VariableName=vgrid_xi_pll_pos  SampleTime=-1
      settings: MaxDataPoints=Ns_afe
  To Workspace6 : ToWorkspace  VariableName=vgrid_eta_pll_pos  SampleTime=-1
      settings: MaxDataPoints=Ns_afe
  Unit Delay1 : UnitDelay  SampleTime=-1  HasFrameUpgradeWarning=on
  Unit Delay2 : UnitDelay  SampleTime=-1  HasFrameUpgradeWarning=on
  Unit Delay4 : UnitDelay  SampleTime=-1  HasFrameUpgradeWarning=on
  bounder1 : MATLAB Function  TreatAsAtomicUnit=on
  double_integrator_observer : Subsystem
  kp : Gain  Gain=pll_i1_ddsrt*ts_afe  SaturateOnIntegerOverflow=on  OutDataTypeStr=Inherit: Same as input  ParamDataTypeStr=Inherit: Same as input
  kp1 : Gain  Gain=pll_p_ddsrt  SaturateOnIntegerOverflow=on  OutDataTypeStr=Inherit: Same as input  ParamDataTypeStr=Inherit: Same as input
  kp2 : Gain  Gain=ts_afe  SaturateOnIntegerOverflow=on  OutDataTypeStr=Inherit: Same as input  ParamDataTypeStr=Inherit: Same as input
  gamma_grid_ddsrf_pll : Outport  VectorParamsAs1DForOutWhenUnconnected=off
  omega_grid_ddsrf_pll : Outport  Port=2  VectorParamsAs1DForOutWhenUnconnected=off
  wires:
  Unit Delay2/1 -> gamma_grid_ddsrf_pll/1, double_integrator_observer/1(theta)
  kp1/1 -> Sum5/1
  Product3/1 -> kp/1, kp1/1  "V l"
  Product2/1 -> kp2/1
  u_grid_pos_eta/1 -> Product1/1, To Workspace6/1
  u_grid_pos_xi/1 -> To Workspace5/1, Product/1
  bounder1/1(y) -> Unit Delay1/1, Unit Delay2/1
  Sum5/1 -> Product2/1
  kp/1 -> Sum3/1
  Switch/1 -> Product3/2
  Sqrt/1 -> Product3/1
  Constant6/1 -> Switch/1
  Constant5/1 -> Switch/3
  [Vgrid_unorm] -> Product1/2, Product/2
  Constant4/1 -> Product2/2
  kp2/1 -> Sum4/1
  -2<x<2/1 -> Unit Delay4/1, Sum5/2  "i1"
  Unit Delay1/1 -> Sum4/2
  Sum4/1 -> bounder1/1(u)
  Sum3/1 -> -2<x<2/1
  Unit Delay4/1 -> Sum3/2
  Sum1/1 -> Math Function2/1, Switch/2
  Sum/1 -> Math Function/1
  Sum2/1 -> Sqrt/1
  Math Function2/1 -> Sum2/2
  Math Function/1 -> Sum2/1
  Constant3/1 -> Sum1/2
  Product1/1 -> Sum1/1
  Constant2/1 -> Sum/2
  Product/1 -> Sum/1
  double_integrator_observer/1(omega_hat) -> omega_grid_ddsrf_pll/1

== system afe_abc_inv_psm_2mods/afe_abc_inv_psm_mod1/AFE_control/afe_control/grid_voltage_phase_lock_loops/dq_pll/pll_stageA ==
  gamma_grid : Inport
  ug_abc : Inport  Port=2
  Demux : Demux  Outputs=3
  Math Function : Math  Operator=magnitude^2  SignedPower=on
  Math Function1 : Math  Operator=magnitude^2  SignedPower=on
  Reciprocal Sqrt : Sqrt  Operator=rSqrt
  Saturation : Saturate  UpperLimit=inf  LowerLimit=0.02
  Sum : Sum  Inputs=|++
  mormalization_and_transformation : Subsystem
  sequences : Subsystem
  u_grid_pos_xi : Outport  VectorParamsAs1DForOutWhenUnconnected=off
  u_grid_pos_eta : Outport  Port=2  VectorParamsAs1DForOutWhenUnconnected=off
  tag scope: Vgrid_unorm_mod1=global
  wires:
  ug_abc/1 -> Demux/1
  Demux/1 -> mormalization_and_transformation/1(ug_a)
  Demux/2 -> mormalization_and_transformation/2(ug_b)
  Demux/3 -> mormalization_and_transformation/3(ug_c)
  gamma_grid/1 -> sequences/3(gamma_grid)
  sequences/1(u_grid_pos_xi) -> u_grid_pos_xi/1
  sequences/2(u_grid_pos_eta) -> u_grid_pos_eta/1
  Math Function1/1 -> Sum/2
  mormalization_and_transformation/1(ug_alpha) -> Math Function/1, sequences/1(u_grid_alpha)
  mormalization_and_transformation/2(ug_beta) -> Math Function1/1, sequences/2(u_grid_beta)
  Reciprocal Sqrt/1 -> [Vgrid_unorm_mod1]
  Sum/1 -> Saturation/1
  Math Function/1 -> Sum/1
  Saturation/1 -> Reciprocal Sqrt/1

== system afe_abc_inv_psm_2mods/afe_abc_inv_psm_mod1/AFE_control/afe_control/grid_voltage_phase_lock_loops/dq_pll/pll_stageB ==
  u_grid_pos_xi : Inport
  u_grid_pos_eta : Inport  Port=2
  -2<x<2 : Saturate  UpperLimit=2  LowerLimit=-2
  Constant4 : Constant  Value=omega_grid_nom
  Product1 : Product  RndMeth=Zero
  Product2 : Product  RndMeth=Zero
  Sum3 : Sum  SaturateOnIntegerOverflow=on
  Sum4 : Sum  SaturateOnIntegerOverflow=on
  Sum5 : Sum  Inputs=++|
  Unit Delay1 : UnitDelay  SampleTime=-1  HasFrameUpgradeWarning=on
  Unit Delay2 : UnitDelay  SampleTime=-1  HasFrameUpgradeWarning=on
  Unit Delay4 : UnitDelay  SampleTime=-1  HasFrameUpgradeWarning=on
  bounder1 : MATLAB Function  TreatAsAtomicUnit=on
  double_integrator_observer : Subsystem
  kp : Gain  Gain=pll_i1*ts_afe  SaturateOnIntegerOverflow=on  OutDataTypeStr=Inherit: Same as input  ParamDataTypeStr=Inherit: Same as input
  kp2 : Gain  Gain=ts_afe  SaturateOnIntegerOverflow=on  OutDataTypeStr=Inherit: Same as input  ParamDataTypeStr=Inherit: Same as input
  scheduled-p-gain : Subsystem
      settings: PortSchema="{\"entries\":[{\"content\":{\"sides\":[{\"content\":{},\"type\":\"ConnectorPlacement.EquallySpacedRectSide\",\"uuid\":\"88e64df2-a299-4c1b-9bac-7a615cd04a00\"},{\"content\":{\"side\":\"RIGHT\"},\"type\":\"ConnectorPlacement.EquallySpacedRectSide\",\"uuid\":\"ef1d7318-b0e2-4e96-bf99-c42bb4ec5202\"},{\"content\":{\"connectorIds\":[\"In1\"],\"side\":\"TOP\"},\"type\":\"ConnectorPlacement.EquallySpacedRectSide\",\"uuid\":\"96582c59-f6c8-40f1-b3cf-394cc239c4b2\"},{\"content\":{\"connectorIds\":[\"Out1\"],\"side\":\"BOTTOM\"},\"type\":\"ConnectorPlacement.EquallySpacedRectSide\",\"uuid\":\"9ac5cd0d-958f-4b67-b4ea-90856a0aa038\"}]},\"type\":\"ConnectorPlacement.EquallySpacedConnector\",\"uuid\":\"ca37db80-6b94-4315-bd9c-66307567cd1f\"}],\"packageUris\":[\"http://schema.mathworks.com/mf0/Connector/R2020b\"],\"version\":\"1.0\"}"
  gamma_grid_pll : Outport  VectorParamsAs1DForOutWhenUnconnected=off
  omega_grid_pll : Outport  Port=2  VectorParamsAs1DForOutWhenUnconnected=off
  wires:
  Unit Delay4/1 -> Sum3/2
  Sum3/1 -> -2<x<2/1
  Sum4/1 -> bounder1/1(u)
  Unit Delay1/1 -> Sum4/2
  -2<x<2/1 -> Sum5/2, Unit Delay4/1  "i1"
  kp2/1 -> Sum4/1
  Constant4/1 -> Product2/2
  [Vgrid_unorm_mod1] -> Product1/2
  kp/1 -> Sum3/1
  Sum5/1 -> Product2/1
  bounder1/1(y) -> Unit Delay1/1, Unit Delay2/1
  u_grid_pos_eta/1 -> Product1/1
  Product2/1 -> kp2/1
  Product1/1 -> scheduled-p-gain/1(In1), kp/1  "V l"
  scheduled-p-gain/1(Out2) -> Sum5/1
  Unit Delay2/1 -> double_integrator_observer/1(theta), gamma_grid_pll/1
  double_integrator_observer/1(omega_hat) -> omega_grid_pll/1
